simulink model "udp_socket"  (R2020b)
settings: Solver=FixedStepAuto  StartTime=0.0  StopTime=inf  FixedStep=0.01  RelTol=1e-3
libraries: slrealtimeutilitieslib x2, simulink x2, dspnetwork x2, sldrtlib x1
settings Model: Creator=maosh  LastModifiedBy=maosh
settings DataIOCC: ReturnWorkspaceOutputs=off
settings OptimizationCC: DefaultParameterBehavior=Inlined  PassReuseOutputArgsThreshold=0
settings DebuggingCC: ParameterTunabilityLossMsg=error  ArithmeticOperatorsInVariantConditions=warning
settings SFSimCC: SimUseLocalCustomCode=off  MATLABDynamicMemAlloc=off  CustomCodeUndefinedFunction=UseInterfaceOnly
settings RTWCC: Description=Simulink Desktop Real-Time  SystemTargetFile=sldrt.tlc  TemplateMakefile=sldrt.tmf  GenerateReport=on  RTWUseLocalCustomCode=off  LaunchReport=on  RTWCompilerOptimization=on
settings CodeAppCC: ForceParamTrailComments=on  MaxIdLength=95  OperatorAnnotations=on
settings SimulinkDesktopRealTimeCC: TargetPreCompLibLocation=D:\MATLAB\RLS2020B\toolbox\sldrt\lib\win64

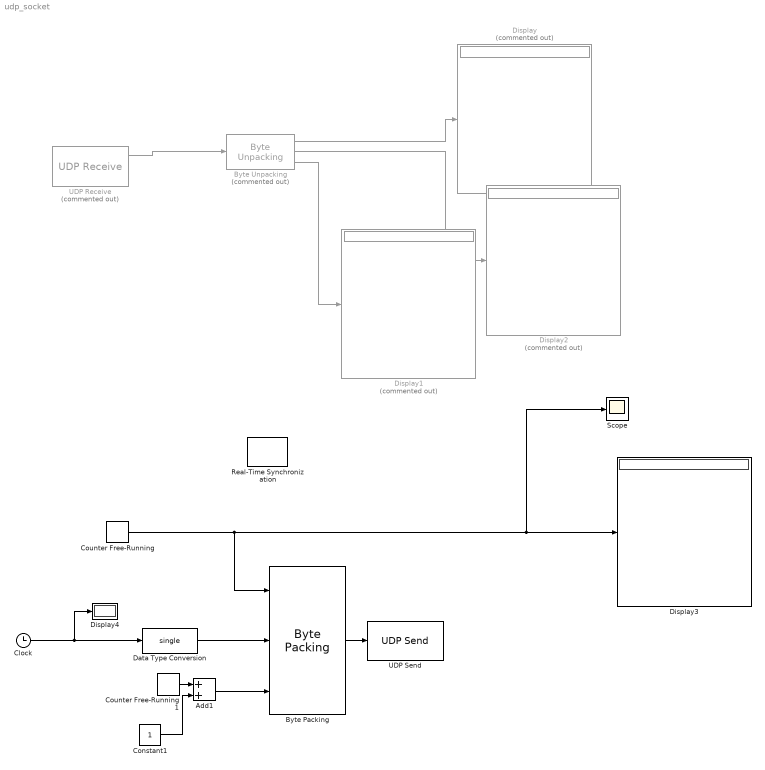
== system udp_socket ==
  Add1 : Sum  OutDataTypeStr=uint32
  "Byte Packing " : slrealtimeutilitieslib/Byte Packing  MaskPackedDataType=uint8  MaskUnpackedDataTypes={'uint32','single','uint32'}  MaskAlignment=1
  "Byte Unpacking " : slrealtimeutilitieslib/Byte Unpacking  Commented=on  MaskUnpackedDataTypes={'uint32','single','uint32'}  MaskUnpackedDataSizes={[1],[1],[1]}  MaskAlignment=1
      settings: SourceProductBaseCode=XP
  Clock : Clock
  Constant1 : Constant
  Counter Free-Running : simulink/Sources/Counter Free-Running  NumBits=32  tsamp=-1
  Counter Free-Running1 : simulink/Sources/Counter Free-Running  NumBits=32  tsamp=-1
  Data Type Conversion : DataTypeConversion  OutDataTypeStr=single
  Display : Display  Commented=on
  Display1 : Display  Commented=on
  Display2 : Display  Commented=on
  Display3 : Display
  Display4 : Display
  Real-Time Synchronization : sldrtlib/Real-Time Synchronization  SampleTime=0.01  MaxMissedTicks=inf  ShowMissedTicks=off  YieldWhenWaiting=off
  Scope : Scope
  UDP Receive : dspnetwork/UDP Receive  Commented=on  localURL='0.0.0.0'  localPort=8888  remoteURL='127.0.0.1'  remotePort=-1  recvBufferSize=8192  dims=12  signalDatatype=uint8  isComplex=off  isVarSize=off  showBlockingTime=off  blockingTime=0  sampletime=1  blockPlatform=[]
  UDP Send : dspnetwork/UDP Send  remoteURL='127.0.0.1'  remotePort=8888  localURL='0.0.0.0'  localPortSource=Automatically determine  localPort=2048  sendBufferSize=8192  sampletime=-1  blockPlatform=[]  separateLengthPort=0
  wires:
  UDP Receive/1 -> "Byte Unpacking "/1
  "Byte Unpacking "/1 -> Display/1
  "Byte Unpacking "/2 -> Display2/1
  "Byte Unpacking "/3 -> Display1/1
  "Byte Packing "/1 -> UDP Send/1
  Counter Free-Running/1 -> "Byte Packing "/1, Scope/1, Display3/1
  Clock/1 -> Data Type Conversion/1, Display4/1
  Counter Free-Running1/1 -> Add1/1
  Add1/1 -> "Byte Packing "/3
  Constant1/1 -> Add1/2
  Data Type Conversion/1 -> "Byte Packing "/2
